simulink model "Pacemaker"  (R2019b)
settings: Solver=FixedStepAuto  StartTime=0.0  StopTime=10.0  FixedStep=1e-3  MaxStep=0.2  RelTol=1e-3  EnableMultiTasking=on
undefined symbols (not defined in the file): D0, D1, D10, D11, D12, D13, D2, D3, D4, D5, D6, D7, D8, D9, PTA0, PTA1, PTA2, PTB23, PTB9, PTC16, PTC17, PTC2, PTC3, PTC4, PTD0, PTD1, PTD2, PTD3
libraries: frdmk64flib x17
settings Model: ExtModeTrigDuration=5  Creator=shahv10  LastModifiedBy=shahv10
settings OptimizationCC: EnhancedBackFolding=on  PassReuseOutputArgsAs=Individual arguments  ZeroExternalMemoryAtStartup=off  ZeroInternalMemoryAtStartup=off  MaxStackSize=64  OptimizeBlockOrder=speed  DifferentSizesBufferReuse=on  OptimizationCustomize=off  EfficientTunableParamExpr=on
settings DebuggingCC: ParameterTunabilityLossMsg=error
settings HardwareCC: ProdBitPerPointer=32  ProdBitPerSizeT=32  ProdBitPerPtrDiffT=32  ProdLargestAtomicInteger=Long  ProdLargestAtomicFloat=Double  ProdWordSize=32  ProdHWDeviceType=ARM Compatible->ARM Cortex  UseEmbeddedCoderFeatures=off
settings SFSimCC: MATLABDynamicMemAlloc=off
settings RTWCC: SystemTargetFile=ert.tlc  HardwareBoard=NXP FRDM-K64F  TLCOptions="-aInlineSetEventsForThisBaseRateFcn=TLC_FALSE -aSuppressMultiTaskScheduler=TLC_FALSE  -aRateBasedStepFcn=0"  TemplateMakefile=ert_default_tmf  GenerateReport=on  Toolchain=GNU Tools for ARM Embedded Processors  IncludeHyperlinkInReport=on  LaunchReport=on  GenerateTraceInfo=on  GenerateTraceReport=on  GenerateTraceReportSl=on  GenerateTraceReportSf=on  GenerateTraceReportEml=on
settings CodeAppCC: ForceParamTrailComments=on  IgnoreCustomStorageClasses=off  OperatorAnnotations=on  SimulinkDataObjDesc=on  SFDataObjDesc=on  InsertBlockDesc=on
settings ERTTargetCC: SupportNonInlinedSFcns=on

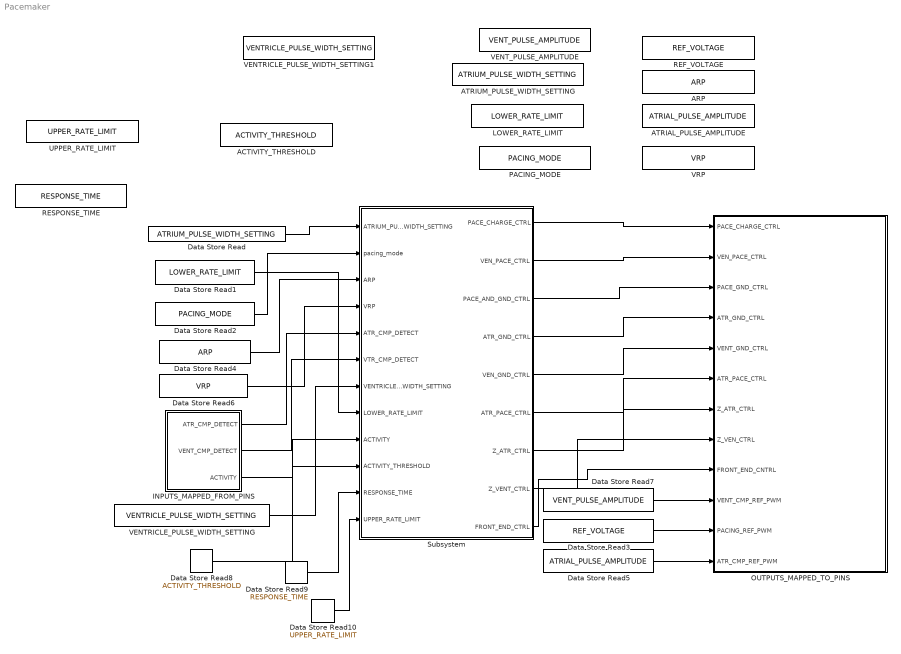
== system Pacemaker ==
  ACTIVITY_THRESHOLD : DataStoreMemory  DataStoreName=ACTIVITY_THRESHOLD  ReadBeforeWriteMsg=warning  WriteAfterWriteMsg=warning  WriteAfterReadMsg=warning  InitialValue=4  ShowAdditionalParam=off  OutDataTypeStr=uint8
  ARP : DataStoreMemory  DataStoreName=ARP  ReadBeforeWriteMsg=warning  WriteAfterWriteMsg=warning  WriteAfterReadMsg=warning  InitialValue=150  ShowAdditionalParam=off  OutDataTypeStr=uint16
  ATRIAL_PULSE_AMPLITUDE : DataStoreMemory  DataStoreName=ATRIAL_PULSE_AMPLITUDE  ReadBeforeWriteMsg=warning  WriteAfterWriteMsg=warning  WriteAfterReadMsg=warning  InitialValue=70  ShowAdditionalParam=off  OutDataTypeStr=uint16
  ATRIUM_PULSE_WIDTH_SETTING : DataStoreMemory  DataStoreName=ATRIUM_PULSE_WIDTH_SETTING  ReadBeforeWriteMsg=warning  WriteAfterWriteMsg=warning  WriteAfterReadMsg=warning  InitialValue=100  ShowAdditionalParam=off  OutDataTypeStr=uint16  Dimensions=1
  Data Store Read : DataStoreRead  DataStoreName=ATRIUM_PULSE_WIDTH_SETTING
  Data Store Read1 : DataStoreRead  DataStoreName=LOWER_RATE_LIMIT
  Data Store Read10 : DataStoreRead  DataStoreName=UPPER_RATE_LIMIT
  Data Store Read2 : DataStoreRead  DataStoreName=PACING_MODE
  Data Store Read3 : DataStoreRead  DataStoreName=REF_VOLTAGE
  Data Store Read4 : DataStoreRead  DataStoreName=ARP
  Data Store Read5 : DataStoreRead  DataStoreName=ATRIAL_PULSE_AMPLITUDE
  Data Store Read6 : DataStoreRead  DataStoreName=VRP
  Data Store Read7 : DataStoreRead  DataStoreName=VENT_PULSE_AMPLITUDE
  Data Store Read8 : DataStoreRead  DataStoreName=ACTIVITY_THRESHOLD
  Data Store Read9 : DataStoreRead  DataStoreName=RESPONSE_TIME
  "INPUTS_MAPPED_FROM_PINS " : Subsystem
  LOWER_RATE_LIMIT : DataStoreMemory  DataStoreName=LOWER_RATE_LIMIT  ReadBeforeWriteMsg=warning  WriteAfterWriteMsg=warning  WriteAfterReadMsg=warning  InitialValue=60  ShowAdditionalParam=off
  "OUTPUTS_MAPPED_TO_PINS " : Subsystem
  PACING_MODE : DataStoreMemory  DataStoreName=PACING_MODE  ReadBeforeWriteMsg=warning  WriteAfterWriteMsg=warning  WriteAfterReadMsg=warning  InitialValue=4  ShowAdditionalParam=off  OutDataTypeStr=uint8
  REF_VOLTAGE : DataStoreMemory  DataStoreName=REF_VOLTAGE  ReadBeforeWriteMsg=warning  WriteAfterWriteMsg=warning  WriteAfterReadMsg=warning  InitialValue=70  ShowAdditionalParam=off  OutDataTypeStr=uint8
  RESPONSE_TIME : DataStoreMemory  DataStoreName=RESPONSE_TIME  ReadBeforeWriteMsg=warning  WriteAfterWriteMsg=warning  WriteAfterReadMsg=warning  InitialValue=4  ShowAdditionalParam=off  OutDataTypeStr=uint8
  Subsystem : Subsystem
  UPPER_RATE_LIMIT : DataStoreMemory  DataStoreName=UPPER_RATE_LIMIT  ReadBeforeWriteMsg=warning  WriteAfterWriteMsg=warning  WriteAfterReadMsg=warning  InitialValue=4  ShowAdditionalParam=off  OutDataTypeStr=uint8
  VENTRICLE_PULSE_WIDTH_SETTING : DataStoreRead  DataStoreName=VENTRICLE_PULSE_WIDTH_SETTING
  VENTRICLE_PULSE_WIDTH_SETTING1 : DataStoreMemory  DataStoreName=VENTRICLE_PULSE_WIDTH_SETTING  ReadBeforeWriteMsg=warning  WriteAfterWriteMsg=warning  WriteAfterReadMsg=warning  InitialValue=20  ShowAdditionalParam=off  OutDataTypeStr=uint16  Dimensions=1
  VENT_PULSE_AMPLITUDE : DataStoreMemory  DataStoreName=VENT_PULSE_AMPLITUDE  ReadBeforeWriteMsg=warning  WriteAfterWriteMsg=warning  WriteAfterReadMsg=warning  InitialValue=70  ShowAdditionalParam=off  OutDataTypeStr=uint16
  VRP : DataStoreMemory  DataStoreName=VRP  ReadBeforeWriteMsg=warning  WriteAfterWriteMsg=warning  WriteAfterReadMsg=warning  InitialValue=150  ShowAdditionalParam=off  OutDataTypeStr=uint16
  wires:
  Subsystem/6(ATR_PACE_CTRL) -> "OUTPUTS_MAPPED_TO_PINS "/6(ATR_PACE_CTRL)
  Subsystem/1("PACE_CHARGE_CTRL ") -> "OUTPUTS_MAPPED_TO_PINS "/1(PACE_CHARGE_CTRL)
  Subsystem/2(VEN_PACE_CTRL) -> "OUTPUTS_MAPPED_TO_PINS "/2(VEN_PACE_CTRL)
  Subsystem/3(PACE_AND_GND_CTRL) -> "OUTPUTS_MAPPED_TO_PINS "/3(PACE_GND_CTRL)
  Subsystem/4("ATR_GND_CTRL ") -> "OUTPUTS_MAPPED_TO_PINS "/4(ATR_GND_CTRL)
  Subsystem/5("VEN_GND_CTRL ") -> "OUTPUTS_MAPPED_TO_PINS "/5(VENT_GND_CTRL)
  Data Store Read/1 -> Subsystem/1(ATRIUM_PULSE_WIDTH_SETTING)
  Data Store Read2/1 -> Subsystem/2(pacing_mode)
  Data Store Read3/1 -> "OUTPUTS_MAPPED_TO_PINS "/11("PACING_REF_PWM ")
  Subsystem/7(Z_ATR_CTRL) -> "OUTPUTS_MAPPED_TO_PINS "/7(Z_ATR_CTRL)
  Subsystem/8(Z_VENT_CTRL) -> "OUTPUTS_MAPPED_TO_PINS "/8(Z_VEN_CTRL)
  Data Store Read4/1 -> Subsystem/3(ARP)
  "INPUTS_MAPPED_FROM_PINS "/1(ATR_CMP_DETECT) -> Subsystem/5(ATR_CMP_DETECT)
  Data Store Read5/1 -> "OUTPUTS_MAPPED_TO_PINS "/12("ATR_CMP_REF_PWM ")
  Subsystem/9(FRONT_END_CTRL) -> "OUTPUTS_MAPPED_TO_PINS "/9(FRONT_END_CNTRL)
  "INPUTS_MAPPED_FROM_PINS "/2(VENT_CMP_DETECT) -> Subsystem/6(VTR_CMP_DETECT)
  Data Store Read6/1 -> Subsystem/4(VRP)
  Data Store Read7/1 -> "OUTPUTS_MAPPED_TO_PINS "/10(VENT_CMP_REF_PWM)
  VENTRICLE_PULSE_WIDTH_SETTING/1 -> Subsystem/7(VENTRICLE_PULSE_WIDTH_SETTING)
  Data Store Read1/1 -> Subsystem/8("LOWER_RATE_LIMIT ")
  "INPUTS_MAPPED_FROM_PINS "/3(ACTIVITY) -> Subsystem/9(ACTIVITY)
  Data Store Read8/1 -> Subsystem/10(ACTIVITY_THRESHOLD)
  Data Store Read9/1 -> Subsystem/11(RESPONSE_TIME)
  Data Store Read10/1 -> Subsystem/12(UPPER_RATE_LIMIT)

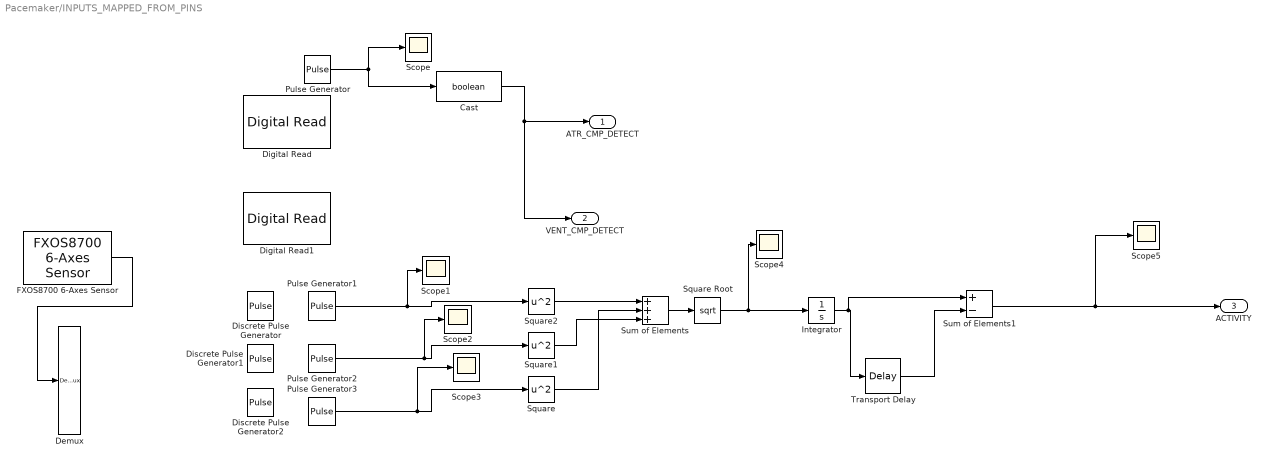
== system Pacemaker/INPUTS_MAPPED_FROM_PINS  ==
  Cast : DataTypeConversion  OutDataTypeStr=boolean
  Demux : Demux  Outputs=3
  Digital Read : frdmk64flib/Digital Read  Whichpin=PTC16 (D0)  SampleTime=-1
      settings: SourceProductName=Simulink Coder Support Package for NXP FRDM-K64F Board
  Digital Read1 : frdmk64flib/Digital Read  Whichpin=PTC17 (D1)  SampleTime=-1
      settings: SourceProductName=Simulink Coder Support Package for NXP FRDM-K64F Board
  Discrete Pulse Generator : DiscretePulseGenerator  Period=10  PulseWidth=5
  Discrete Pulse Generator1 : DiscretePulseGenerator  Amplitude=2  Period=10  PulseWidth=5  PhaseDelay=2
  Discrete Pulse Generator2 : DiscretePulseGenerator  Amplitude=3  Period=10  PulseWidth=5  PhaseDelay=4
  FXOS8700 6-Axes Sensor : frdmk64flib/FXOS8700 6-Axes Sensor  Activesensor=Accelerometer only  ODR=800Hz  HybridODR=400Hz  Accelfullrange=-4g to +4g  SampleTime=-1
      settings: SourceProductName=Simulink Coder Support Package for NXP FRDM-K64F Board
  Integrator : Integrator
  Pulse Generator : DiscretePulseGenerator  PulseType=Time based  Period=1.3  PulseWidth=5  PhaseDelay=1
  Pulse Generator1 : DiscretePulseGenerator  PulseType=Time based  Period=10  PulseWidth=50
  Pulse Generator2 : DiscretePulseGenerator  PulseType=Time based  Amplitude=2  Period=10  PulseWidth=50  PhaseDelay=2  VectorParams1D=off
  Pulse Generator3 : DiscretePulseGenerator  PulseType=Time based  Amplitude=3  Period=10  PulseWidth=50  PhaseDelay=4
  Scope{,1..5} (6 alike) : Scope
  Square : Math  Operator=square  SignedPower=off  SaturateOnIntegerOverflow=on
  Square Root : Sqrt  SaturateOnIntegerOverflow=on
  Square1 : Math  Operator=square  SignedPower=off  SaturateOnIntegerOverflow=on
  Square2 : Math  Operator=square  SignedPower=off  SaturateOnIntegerOverflow=on
  Sum of Elements : Sum  Inputs=+++
  Sum of Elements1 : Sum  Inputs=+-
  Transport Delay : TransportDelay  BufferSize=2048
  ATR_CMP_DETECT : Outport  OutDataTypeStr=boolean
  VENT_CMP_DETECT : Outport  Port=2
  ACTIVITY : Outport  Port=3
  wires:
  Pulse Generator/1 -> Cast/1, Scope/1
  Cast/1 -> ATR_CMP_DETECT/1, VENT_CMP_DETECT/1
  Sum of Elements/1 -> Square Root/1
  Square2/1 -> Sum of Elements/1
  Square1/1 -> Sum of Elements/3
  Square/1 -> Sum of Elements/2
  Square Root/1 -> Integrator/1, Scope4/1
  Sum of Elements1/1 -> Scope5/1, ACTIVITY/1
  Integrator/1 -> Sum of Elements1/1, Transport Delay/1
  Transport Delay/1 -> Sum of Elements1/2
  Pulse Generator3/1 -> Scope3/1, Square/1
  Pulse Generator2/1 -> Scope2/1, Square1/1
  FXOS8700 6-Axes Sensor/1 -> Demux/1
  Pulse Generator1/1 -> Scope1/1, Square2/1

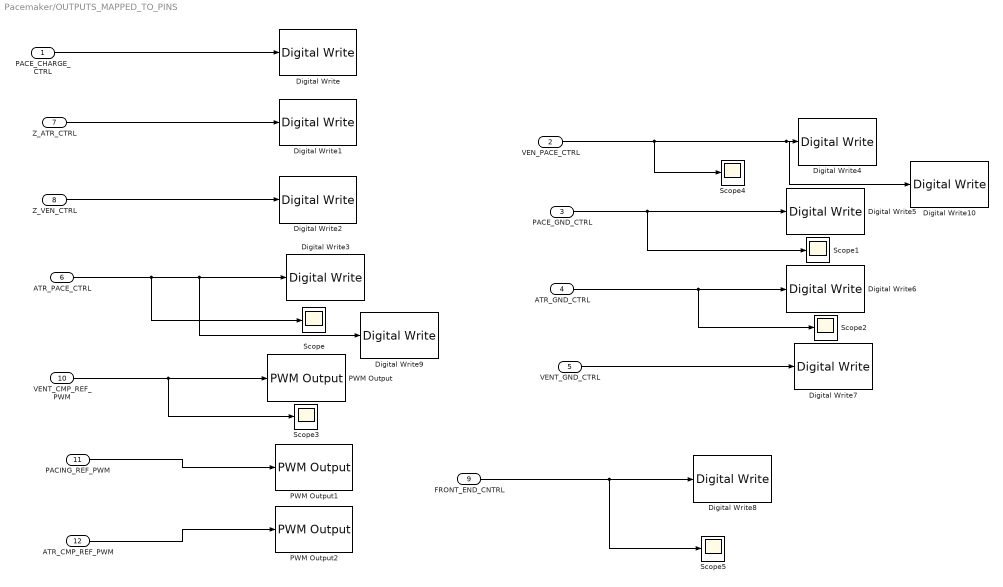
== system Pacemaker/OUTPUTS_MAPPED_TO_PINS  ==
  PACE_CHARGE_CTRL : Inport
  VEN_PACE_CTRL : Inport  Port=2
  PACE_GND_CTRL : Inport  Port=3
  ATR_GND_CTRL : Inport  Port=4
  VENT_GND_CTRL : Inport  Port=5
  ATR_PACE_CTRL : Inport  Port=6
  Z_ATR_CTRL : Inport  Port=7
  Z_VEN_CTRL : Inport  Port=8
  FRONT_END_CNTRL : Inport  Port=9
  VENT_CMP_REF_PWM : Inport  Port=10
  "PACING_REF_PWM " : Inport  Port=11
  "ATR_CMP_REF_PWM " : Inport  Port=12
  Digital Write : frdmk64flib/Digital Write  Whichpin=PTB9 (D2)
      settings: SourceProductName=Simulink Coder Support Package for NXP FRDM-K64F Board
  Digital Write1 : frdmk64flib/Digital Write  Whichpin=PTB23 (D4)
      settings: SourceProductName=Simulink Coder Support Package for NXP FRDM-K64F Board
  Digital Write10 : frdmk64flib/Digital Write  Whichpin=BLUE_LED
      settings: SourceProductName=Simulink Coder Support Package for NXP FRDM-K64F Board
  Digital Write2 : frdmk64flib/Digital Write  Whichpin=PTC3 (D7)
      settings: SourceProductName=Simulink Coder Support Package for NXP FRDM-K64F Board
  Digital Write3 : frdmk64flib/Digital Write  Whichpin=PTA0 (D8)
      settings: SourceProductName=Simulink Coder Support Package for NXP FRDM-K64F Board
  Digital Write4 : frdmk64flib/Digital Write  Whichpin=PTC4 (D9)
      settings: SourceProductName=Simulink Coder Support Package for NXP FRDM-K64F Board
  Digital Write5 : frdmk64flib/Digital Write  Whichpin=PTD0 (D10)
      settings: SourceProductName=Simulink Coder Support Package for NXP FRDM-K64F Board
  Digital Write6 : frdmk64flib/Digital Write  Whichpin=PTD2 (D11)
      settings: SourceProductName=Simulink Coder Support Package for NXP FRDM-K64F Board
  Digital Write7 : frdmk64flib/Digital Write  Whichpin=PTD3 (D12)
      settings: SourceProductName=Simulink Coder Support Package for NXP FRDM-K64F Board
  Digital Write8 : frdmk64flib/Digital Write  Whichpin=PTD1 (D13)
      settings: SourceProductName=Simulink Coder Support Package for NXP FRDM-K64F Board
  Digital Write9 : frdmk64flib/Digital Write  Whichpin=RED_LED
      settings: SourceProductName=Simulink Coder Support Package for NXP FRDM-K64F Board
  PWM Output : frdmk64flib/PWM Output  Whichpin=PTA1 (D3)  InitialFrequency=2000  InitialDutyCycle=0
      settings: SourceProductName=Simulink Coder Support Package for NXP FRDM-K64F Board
  PWM Output1 : frdmk64flib/PWM Output  Whichpin=PTA2 (D5)  InitialFrequency=2000  InitialDutyCycle=0
      settings: SourceProductName=Simulink Coder Support Package for NXP FRDM-K64F Board
  PWM Output2 : frdmk64flib/PWM Output  Whichpin=PTC2 (D6)  InitialFrequency=2000  InitialDutyCycle=0
      settings: SourceProductName=Simulink Coder Support Package for NXP FRDM-K64F Board
  Scope{,1..5} (6 alike) : Scope
  wires:
  PACE_CHARGE_CTRL/1 -> Digital Write/1
  Z_ATR_CTRL/1 -> Digital Write1/1
  Z_VEN_CTRL/1 -> Digital Write2/1
  ATR_PACE_CTRL/1 -> Scope/1, Digital Write9/1, Digital Write3/1
  VENT_GND_CTRL/1 -> Digital Write7/1
  VEN_PACE_CTRL/1 -> Scope4/1, Digital Write10/1, Digital Write4/1
  ATR_GND_CTRL/1 -> Scope2/1, Digital Write6/1
  PACE_GND_CTRL/1 -> Scope1/1, Digital Write5/1
  FRONT_END_CNTRL/1 -> Scope5/1, Digital Write8/1
  VENT_CMP_REF_PWM/1 -> Scope3/1, PWM Output/1
  "PACING_REF_PWM "/1 -> PWM Output1/1
  "ATR_CMP_REF_PWM "/1 -> PWM Output2/1

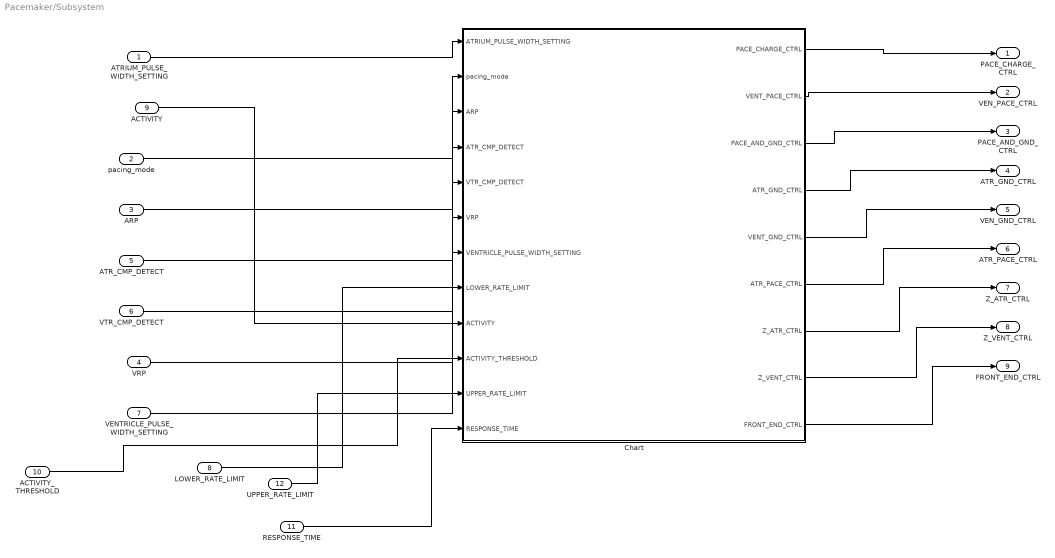
== system Pacemaker/Subsystem ==
  ATRIUM_PULSE_WIDTH_SETTING : Inport  OutDataTypeStr=uint16
  pacing_mode : Inport  Port=2  OutDataTypeStr=uint8
  ARP : Inport  Port=3  OutDataTypeStr=uint16
  VRP : Inport  Port=4
  ATR_CMP_DETECT : Inport  Port=5  OutDataTypeStr=boolean
  VTR_CMP_DETECT : Inport  Port=6
  VENTRICLE_PULSE_WIDTH_SETTING : Inport  Port=7  OutDataTypeStr=uint16
  "LOWER_RATE_LIMIT " : Inport  Port=8
  ACTIVITY : Inport  Port=9
  ACTIVITY_THRESHOLD : Inport  Port=10
  RESPONSE_TIME : Inport  Port=11
  UPPER_RATE_LIMIT : Inport  Port=12
  Chart : Stateflow chart  BlockKeywords=__PRM__SERIALIZED__DATA__:Stateflow Chart,Stateflow Diagram  TreatAsAtomicUnit=on
  "PACE_CHARGE_CTRL " : Outport
  VEN_PACE_CTRL : Outport  Port=2
  PACE_AND_GND_CTRL : Outport  Port=3
  "ATR_GND_CTRL " : Outport  Port=4
  "VEN_GND_CTRL " : Outport  Port=5
  ATR_PACE_CTRL : Outport  Port=6
  Z_ATR_CTRL : Outport  Port=7
  Z_VENT_CTRL : Outport  Port=8
  FRONT_END_CTRL : Outport  Port=9
  wires:
  ATRIUM_PULSE_WIDTH_SETTING/1 -> Chart/1(ATRIUM_PULSE_WIDTH_SETTING)
  Chart/1(PACE_CHARGE_CTRL) -> "PACE_CHARGE_CTRL "/1
  Chart/2(VENT_PACE_CTRL) -> VEN_PACE_CTRL/1
  Chart/3(PACE_AND_GND_CTRL) -> PACE_AND_GND_CTRL/1
  Chart/4(ATR_GND_CTRL) -> "ATR_GND_CTRL "/1
  Chart/6(ATR_PACE_CTRL) -> ATR_PACE_CTRL/1
  Chart/5(VENT_GND_CTRL) -> "VEN_GND_CTRL "/1
  pacing_mode/1 -> Chart/2(pacing_mode)
  Chart/7(Z_ATR_CTRL) -> Z_ATR_CTRL/1
  Chart/8(Z_VENT_CTRL) -> Z_VENT_CTRL/1
  ARP/1 -> Chart/3(ARP)
  Chart/9(FRONT_END_CTRL) -> FRONT_END_CTRL/1
  ATR_CMP_DETECT/1 -> Chart/4(ATR_CMP_DETECT)
  VTR_CMP_DETECT/1 -> Chart/5(VTR_CMP_DETECT)
  VRP/1 -> Chart/6(VRP)
  VENTRICLE_PULSE_WIDTH_SETTING/1 -> Chart/7(VENTRICLE_PULSE_WIDTH_SETTING)
  "LOWER_RATE_LIMIT "/1 -> Chart/8(LOWER_RATE_LIMIT)
  ACTIVITY/1 -> Chart/9(ACTIVITY)
  ACTIVITY_THRESHOLD/1 -> Chart/10(ACTIVITY_THRESHOLD)
  RESPONSE_TIME/1 -> Chart/12(RESPONSE_TIME)
  UPPER_RATE_LIMIT/1 -> Chart/11(UPPER_RATE_LIMIT)

== stateflow chart Pacemaker/Subsystem/Chart ==
  state Rate_Sensing
    (default) -> (junction 346) : {counter = 0}
    (junction 330) -> (junction 346) : {counter = counter + 1}
    (junction 343) -> (junction 346) : {counter = 0}
    (junction 346) -> (junction 328)
    (junction 328) -> (junction 343) [order 2] : [ACTIVITY< ACTIVITY_THRESHOLD]
    (junction 328) -> (junction 330) [order 1] : [ACTIVITY >= ACTIVITY_THRESHOLD]
    (junction 328) -> (junction 350) [order 3] : after(1/(CURRENT_RATE_LIMIT/60)*1000 - TOTAL_PULSE_WIDTH,msec)
    (junction 371) -> (junction 376) : {CURRENT_RATE_LIMIT=min(CURRENT_RATE_LIMIT, UPPER_RATE_LIMIT)}
    (junction 350) -> (junction 356) [order 1] : [counter == 1/(CURRENT_RATE_LIMIT/60)*1000 - TOTAL_PULSE_WIDTH]
    (junction 356) -> (junction 360) : {master_counter = master_counter + 1}
    (junction 360) -> (junction 364) [order 1] : [master_counter >= LOWER_RATE_LIMIT/6]
    (junction 364) -> (junction 371) : {CURRENT_RATE_LIMIT = CURRENT_RATE_LIMIT + (UPPER_RATE_LIMIT-LOWER_RATE_LIMIT)/RESPONSE_TIME}
    (junction 376) -> ?
    (junction 360) -> (junction 376) [order 2]
    (junction 350) -> (junction 381) [order 2] : [counter == -1/(CURRENT_RATE_LIMIT/60)*1000 - TOTAL_PULSE_WIDTH]
    (junction 381) -> (junction 376) : {master_counter =0}
  state Atrium_Sense
    state Entry_state
      entry:
      time_wait=(1/(LOWER_RATE_LIMIT/60))*1000 - ARP-ATRIUM_PULSE_WIDTH_SETTING;
    state Exit_state
      entry:
      FRONT_END_CTRL=false;
    (default) -> Atrium_Sense.Entry_state : {FRONT_END_CTRL=true; }
    Atrium_Sense.Entry_state -> (junction 273) [order 1] : [ATR_CMP_DETECT == true ]
    (junction 273) -> Atrium_Sense.Exit_state : {ATR_SENSED=true}
    Atrium_Sense.Entry_state -> Atrium_Sense.Exit_state [order 2] : after(time_wait,msec)
  state Atrium_Pace
    state PaceOff
      entry:
      ATR_PACE_CTRL=false;
      PACE_CHARGE_CTRL=true;
      VENT_PACE_CTRL=false;
      PACE_AND_GND_CTRL=true;
      ATR_GND_CTRL=true;
      VENT_GND_CTRL=false;
      Z_ATR_CTRL=false;
      Z_VENT_CTRL=false;
      TOTAL_PULSE_WIDTH = TOTAL_PULSE_WIDTH + ATRIUM_PULSE_WIDTH_SETTING
    state PaceOn
      entry:
      PACE_CHARGE_CTRL=false;
      ATR_PACE_CTRL=true;
      VENT_PACE_CTRL=false;
      PACE_AND_GND_CTRL=true;
      ATR_GND_CTRL=false;
      VENT_GND_CTRL=false;
      Z_ATR_CTRL=false;
      Z_VENT_CTRL=false;
    (default) -> Atrium_Pace.PaceOn
    Atrium_Pace.PaceOn -> Atrium_Pace.PaceOff : after(ATRIUM_PULSE_WIDTH_SETTING,msec)
  state Ventricle_sense
    state Entry_state
      entry:
      time_wait=(1/(LOWER_RATE_LIMIT/60))*1000 - VRP - VENTRICLE_PULSE_WIDTH_SETTING;
    state Exit_state
      entry:
      FRONT_END_CTRL=false;
    (default) -> Ventricle_sense.Entry_state : {FRONT_END_CTRL=true; }
    Ventricle_sense.Entry_state -> (junction 260) [order 1] : [VTR_CMP_DETECT == true ]
    (junction 260) -> Ventricle_sense.Exit_state : {VENT_SENSED=true}
    Ventricle_sense.Entry_state -> Ventricle_sense.Exit_state [order 2] : after(time_wait,msec)
  state Ventricle_Pace
    state PaceOn
      entry:
      PACE_CHARGE_CTRL=false;
      ATR_PACE_CTRL=false;
      VENT_PACE_CTRL=true;
      PACE_AND_GND_CTRL=true;
      ATR_GND_CTRL=false;
      VENT_GND_CTRL=false;
      Z_ATR_CTRL=false;
      Z_VENT_CTRL=false;
    state PaceOff
      entry:
      ATR_PACE_CTRL=false;
      PACE_CHARGE_CTRL=true;
      VENT_PACE_CTRL=false;
      PACE_AND_GND_CTRL=true;
      ATR_GND_CTRL=false;
      VENT_GND_CTRL=true;
      Z_ATR_CTRL=false;
      Z_VENT_CTRL=false;
      TOTAL_PULSE_WIDTH = TOTAL_PULSE_WIDTH + VENTRICLE_PULSE_WIDTH_SETTING
    (default) -> Ventricle_Pace.PaceOn
    Ventricle_Pace.PaceOn -> Ventricle_Pace.PaceOff : after(VENTRICLE_PULSE_WIDTH_SETTING,msec)
  state DO_NOTHING
  Atrium_Pace.PaceOff -> (junction 300)
  Ventricle_Pace.PaceOff -> (junction 74)
  Ventricle_sense.Exit_state -> (junction 243)
  Atrium_Sense.Exit_state -> (junction 118)
  (junction 69) -> Rate_Sensing [order 2] : [pacing_mode == 5 || pacing_mode ==6 || pacing_mode == 9 ]
  (junction 254) -> (junction 255) : after(ATRIUM_PULSE_WIDTH_SETTING,msec)
  (junction 255) -> (junction 3)
  (junction 118) -> (junction 254) [order 1] : [ATR_SENSED== true]
  (junction 308) -> (junction 289) : after(1/(LOWER_RATE_LIMIT/60)*1000 - TOTAL_PULSE_WIDTH,msec)
  (junction 69) -> (junction 308) [order 1] : [pacing_mode>=0 && pacing_mode<=4]
  (junction 289) -> (junction 3) : {TOTAL_PULSE_WIDTH = 0}
  (junction 67) -> (junction 69) [order 1] : [pacing_mode ==0 || pacing_mode == 1|| pacing_mode ==4]
  (default) -> (junction 257) : {TOTAL_PULSE_WIDTH = 0; CURRENT_RATE_LIMIT=LOWER_RATE_LIMIT}
  (junction 250) -> (junction 251)
  (junction 118) -> (junction 250) [order 2] : [ATR_SENSED == false]
  (junction 251) -> Atrium_Pace
  (junction 300) -> (junction 67) [order 2]
  (junction 67) -> (junction 105) [order 2] : [pacing_mode == 2]
  (junction 105) -> (junction 270) : after(ARP, msec)
  (junction 270) -> Atrium_Sense : {ATR_SENSED=false;}
  (junction 67) -> (junction 236) [order 3] : [pacing_mode == 3]
  (junction 300) -> Ventricle_Pace [order 1] : [pacing_mode == 4]
  (junction 74) -> (junction 67)
  (junction 257) -> (junction 3)
  (junction 3) -> Atrium_Pace [order 1] : [pacing_mode == 0 || pacing_mode ==4]
  (junction 283) -> (junction 3)
  (junction 3) -> (junction 27) [order 2]
  (junction 27) -> Ventricle_Pace [order 1] : [pacing_mode == 1]
  (junction 79) -> (junction 74)
  (junction 27) -> (junction 31) [order 2]
  (junction 236) -> (junction 265) : after(VRP,msec)
  (junction 265) -> Ventricle_sense : {VENT_SENSED=false;}
  (junction 243) -> (junction 280) [order 2]
  (junction 243) -> (junction 282) [order 1] : [VENT_SENSED == true]
  (junction 280) -> Ventricle_Pace : [VENT_SENSED==false]
  DO_NOTHING -> (junction 79)
  (junction 31) -> DO_NOTHING
  (junction 282) -> (junction 283) : after(VENTRICLE_PULSE_WIDTH_SETTING,msec)
  data: ATRIUM_PULSE_WIDTH_SETTING input uint16 size=1; PACE_CHARGE_CTRL output boolean size=1; VENT_PACE_CTRL output boolean size=1; PACE_AND_GND_CTRL output boolean size=1; ATR_GND_CTRL output boolean size=1; VENT_GND_CTRL output boolean size=1; ATR_PACE_CTRL output; pacing_mode input uint8; Z_ATR_CTRL output; Z_VENT_CTRL output; ARP input uint16; FRONT_END_CTRL output boolean; ATR_CMP_DETECT input boolean; time_wait local; VTR_CMP_DETECT input; VRP input; ATR_SENSED local; VENT_SENSED local; VENTRICLE_PULSE_WIDTH_SETTING input uint16; TOTAL_PULSE_WIDTH local uint16; LOWER_RATE_LIMIT input; ACTIVITY input; ACTIVITY_THRESHOLD input; counter local; CURRENT_RATE_LIMIT local; UPPER_RATE_LIMIT input; RESPONSE_TIME input; master_counter local
